simulink model "model_pert"  (R2021a)
settings: Solver=FixedStepAuto  StartTime=0.0  StopTime=2  FixedStep=step  RelTol=1e-3
values from neighbouring files (symbols this model uses):
  Kp = (wn^2) * eye(2)    [TP.m]
  Kv = 2*sqrt(Kp)    [TP.m]
  qc = robot.ikine(Tcart,q0,'mask',mask)    [TP.m]
libraries: roblocks x7, simulink x2
settings Model: Creator=ohvic  LastModifiedBy=ohvic

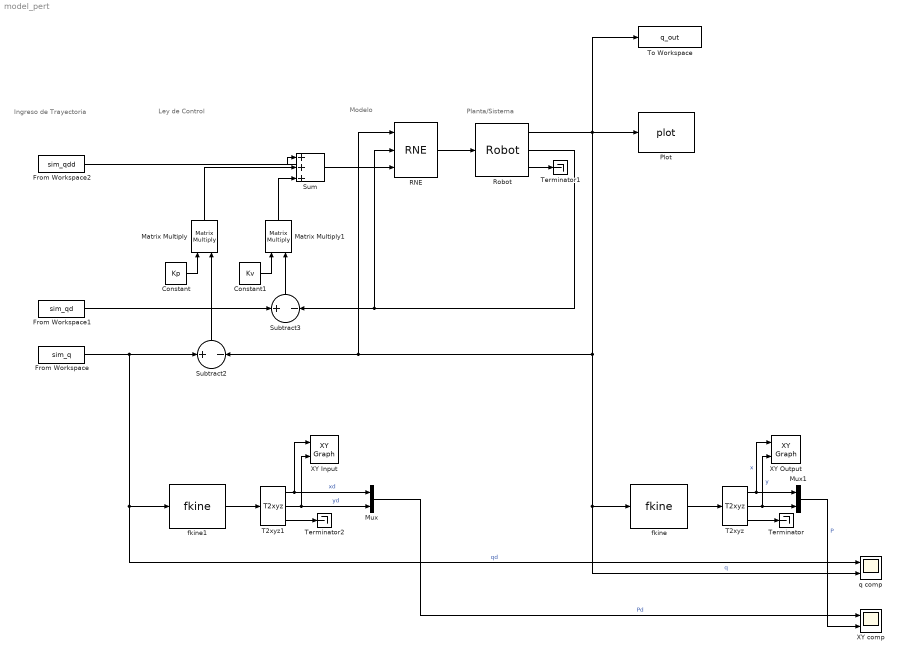
== system model_pert ==
  note: Planta/Sistema
  note: Modelo
  note: Ley de Control
  note: Ingreso de Trayectoria
  Constant : Constant  Value=Kp
  Constant1 : Constant  Value=Kv
  From Workspace : FromWorkspace  VariableName=sim_q  SampleTime=step
  From Workspace1 : FromWorkspace  VariableName=sim_qd  SampleTime=step
  From Workspace2 : FromWorkspace  VariableName=sim_qdd  SampleTime=step
  Matrix Multiply : Product  Multiplication=Matrix(*)
  Matrix Multiply1 : Product  Multiplication=Matrix(*)
  Mux : Mux  Inputs=2
  Mux1 : Mux  Inputs=2
  Plot : roblocks/Arm/plot  robot=robot_dis  fps=25  holdplot=on
  RNE : roblocks/Arm/RNE  robot=robot_dis  grav=[0 0 9.81]
  Robot : roblocks/Arm/Robot  robot=robot_dis  q0=qc(1,:)
  Subtract2 : Sum  Inputs=+-
  Subtract3 : Sum  Inputs=+-
  Sum : Sum  Inputs=|+++
  T2xyz : roblocks/Toolbox/T2xyz
  T2xyz1 : roblocks/Toolbox/T2xyz
  Terminator : Terminator
  Terminator1 : Terminator
  Terminator2 : Terminator
  To Workspace : ToWorkspace  VariableName=q_out  SaveFormat=Timeseries  SampleTime=-1
  XY Input : simulink/Sinks/XY Graph  xmin=-2  xmax=2  ymin=-2  ymax=2  st=-1
  XY Output : simulink/Sinks/XY Graph  xmin=-2  xmax=2  ymin=-2  ymax=2  st=-1
  XY comp : Scope  NumInputPorts=2
  fkine : roblocks/Arm/fkine  robot=robot_dis
  fkine1 : roblocks/Arm/fkine  robot=robot_dis
  q comp : Scope  NumInputPorts=2
  wires:
  Constant/1 -> Matrix Multiply/1
  Constant1/1 -> Matrix Multiply1/1
  From Workspace1/1 -> Subtract3/1
  Subtract2/1 -> Matrix Multiply/2
  Subtract3/1 -> Matrix Multiply1/2
  From Workspace2/1 -> Sum/1
  Matrix Multiply/1 -> Sum/2
  Matrix Multiply1/1 -> Sum/3
  Robot/3 -> Terminator1/1
  T2xyz/1 -> XY Output/1, Mux1/1  "x"
  T2xyz/2 -> Mux1/2, XY Output/2  "y"
  fkine/1 -> T2xyz/1
  T2xyz/3 -> Terminator/1
  Robot/2 -> Subtract3/2, RNE/2
  Robot/1 -> To Workspace/1, fkine/1, q comp/2, Subtract2/2, RNE/1, Plot/1  "q"
  Sum/1 -> RNE/3
  RNE/1 -> Robot/1
  T2xyz1/3 -> Terminator2/1
  T2xyz1/1 -> XY Input/1, Mux/1  "xd"
  fkine1/1 -> T2xyz1/1
  T2xyz1/2 -> XY Input/2, Mux/2  "yd"
  From Workspace/1 -> Subtract2/1, q comp/1, fkine1/1  "qd"
  Mux/1 -> XY comp/1  "Pd"
  Mux1/1 -> XY comp/2  "P"
